simulink model "Sim_8Bus_Chain"  (R2020b)
settings: Solver=FixedStepAuto  StartTime=0  StopTime=3  FixedStep=Ts  RelTol=1e-3
values from neighbouring files (symbols this model uses):
  OtherInputs =     [matlab.mat]
  Ts = 1/Fs    [Main.m]    (also in main.m; matlab.mat = 3.33333333333e-05)
  Wbase = data.basic.Fbase*2*pi    [ConvertExcelFiles.m]    (also in Main.m = Fbase*2*pi; convertExcelFiles.m; main.m = W0; matlab.mat = 376.991118431)
  x_e =     [matlab.mat]
  Zbase = Sbase/Ibase    [Main.m]    (also in matlab.mat = 1e-09)
undefined symbols (not defined in the file or in its folder): DeviceDiscreDamping, DevicePara, DevicePowerFlow, DeviceType
libraries: powerlib x25, SimplexPS x24
settings Model: Creator=admin_user  LastModifiedBy=admin_user

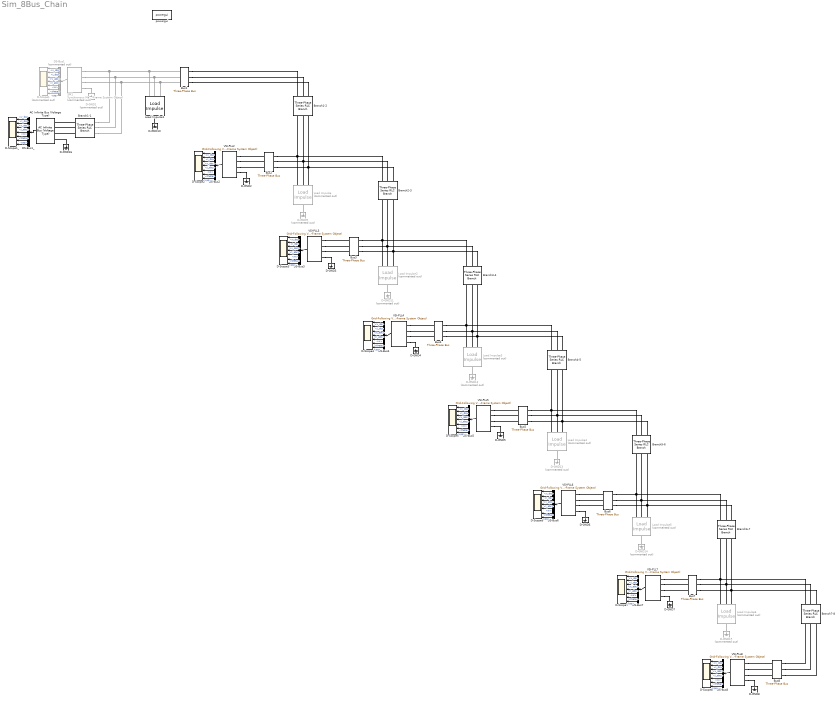
== system Sim_8Bus_Chain ==
  AC Infinite Bus (Voltage Type) : SimplexPS/AC Infinite Bus (Voltage Type)  Ts=Ts  Sbase=Sbase  Vbase=Vbase  Wbase=Wbase  vd=1  vq=0  theta0=0  w=Wbase  R=1e-30
  Branch1-1 : powerlib/Elements/Three-Phase Series RLC Branch  LConnTagsString=A|B|C  RConnTagsString=A|B|C  BranchType=RL  Resistance=(0.001)*Zbase  Inductance=(0.05)*Zbase/Wbase  Capacitance=1e-6  Measurements=None
  Branch1-2 : powerlib/Elements/Three-Phase Series RLC Branch  LConnTagsString=A|B|C  RConnTagsString=A|B|C  BranchType=RL  Resistance=(0.015)*Zbase  Inductance=(0.15)*Zbase/Wbase  Capacitance=1e-6  Measurements=None
  Branch2-3 : powerlib/Elements/Three-Phase Series RLC Branch  LConnTagsString=A|B|C  RConnTagsString=A|B|C  BranchType=RL  Resistance=(0.015)*Zbase  Inductance=(0.15)*Zbase/Wbase  Capacitance=1e-6  Measurements=None
  Branch3-4 : powerlib/Elements/Three-Phase Series RLC Branch  LConnTagsString=A|B|C  RConnTagsString=A|B|C  BranchType=RL  Resistance=(0.015)*Zbase  Inductance=(0.15)*Zbase/Wbase  Capacitance=1e-6  Measurements=None
  Branch4-5 : powerlib/Elements/Three-Phase Series RLC Branch  LConnTagsString=A|B|C  RConnTagsString=A|B|C  BranchType=RL  Resistance=(0.015)*Zbase  Inductance=(0.15)*Zbase/Wbase  Capacitance=1e-6  Measurements=None
  Branch5-6 : powerlib/Elements/Three-Phase Series RLC Branch  LConnTagsString=A|B|C  RConnTagsString=A|B|C  BranchType=RL  Resistance=(0.015)*Zbase  Inductance=(0.15)*Zbase/Wbase  Capacitance=1e-6  Measurements=None
  Branch6-7 : powerlib/Elements/Three-Phase Series RLC Branch  LConnTagsString=A|B|C  RConnTagsString=A|B|C  BranchType=RL  Resistance=(0.015)*Zbase  Inductance=(0.15)*Zbase/Wbase  Capacitance=1e-6  Measurements=None
  Branch7-8 : powerlib/Elements/Three-Phase Series RLC Branch  LConnTagsString=A|B|C  RConnTagsString=A|B|C  BranchType=RL  Resistance=(0.015)*Zbase  Inductance=(0.15)*Zbase/Wbase  Capacitance=1e-6  Measurements=None
  Bus{1..8} (8 alike) : SimplexPS/Three-Phase Bus  Vbase=1  Sbase=1
  D-GND{1,9,11..15} (7 alike) : powerlib/Elements/Ground  Commented=on  LConnTagsString=a
  D-GND{2..8,10,16} (9 alike) : powerlib/Elements/Ground  LConnTagsString=a
  D-Scope1 : Scope  Commented=on  NumInputPorts=7
  D-Scope1_ : Scope  NumInputPorts=7
  D-Scope{2..8} (7 alike) : Scope  NumInputPorts=7
  DS-Bus1 : BusSelector  Commented=on  OutputSignals=v_dq,i_dq,v_abc,i_abc,w,theta,pq
  DS-Bus1_ : BusSelector  OutputSignals=v_dq,i_dq,v_abc,i_abc,w,theta,pq
  DS-Bus{2..8} (7 alike) : BusSelector  OutputSignals=v_dq,i_dq,v_abc,i_abc,w,theta,pq
  Load Impulse{,2..6} (6 alike) : SimplexPS/Load Impulse  Commented=on  t0=1  dt=1/60*4  R=1e-9*Zbase
  Load Impulse1 : SimplexPS/Load Impulse  t0=1  dt=1/60*4  R=1e-9*Zbase
  SM1 : SimplexPS/Synchronous Machine (dq-Frame System Object)  Commented=on  Ts=Ts  Sbase=Sbase  Vbase=Vbase  Wbase=Wbase  DeviceType=DeviceType{1}  DevicePara=DevicePara{1}  PowerFlow=DevicePowerFlow{1}  x0=x_e{1}  OtherInputs=OtherInputs{1}  DiscreMethod=Hybrid Trapezoidal  EnableInsideModification=off  DiscreDampingFlag=on  DiscreDampingValue=DeviceDiscreDamping{1}  LinearizationTimes=1  DirectFeedthrough=off
  VSI-PLL2 : SimplexPS/Grid-Following Voltage-Source Inverter (dq-Frame System Object)  Ts=Ts  Sbase=Sbase  Vbase=Vbase  Wbase=Wbase  DeviceType=DeviceType{2}  DevicePara=DevicePara{2}  PowerFlow=DevicePowerFlow{2}  x0=x_e{2}  OtherInputs=OtherInputs{2}  DiscreMethod=Hybrid Trapezoidal  EnableInsideModification=off  DiscreDampingFlag=on  DiscreDampingValue=DeviceDiscreDamping{2}  LinearizationTimes=1  DirectFeedthrough=off
  VSI-PLL3 : SimplexPS/Grid-Following Voltage-Source Inverter (dq-Frame System Object)  Ts=Ts  Sbase=Sbase  Vbase=Vbase  Wbase=Wbase  DeviceType=DeviceType{3}  DevicePara=DevicePara{3}  PowerFlow=DevicePowerFlow{3}  x0=x_e{3}  OtherInputs=OtherInputs{3}  DiscreMethod=Hybrid Trapezoidal  EnableInsideModification=off  DiscreDampingFlag=on  DiscreDampingValue=DeviceDiscreDamping{3}  LinearizationTimes=1  DirectFeedthrough=off
  VSI-PLL4 : SimplexPS/Grid-Following Voltage-Source Inverter (dq-Frame System Object)  Ts=Ts  Sbase=Sbase  Vbase=Vbase  Wbase=Wbase  DeviceType=DeviceType{4}  DevicePara=DevicePara{4}  PowerFlow=DevicePowerFlow{4}  x0=x_e{4}  OtherInputs=OtherInputs{4}  DiscreMethod=Hybrid Trapezoidal  EnableInsideModification=off  DiscreDampingFlag=on  DiscreDampingValue=DeviceDiscreDamping{4}  LinearizationTimes=1  DirectFeedthrough=off
  VSI-PLL5 : SimplexPS/Grid-Following Voltage-Source Inverter (dq-Frame System Object)  Ts=Ts  Sbase=Sbase  Vbase=Vbase  Wbase=Wbase  DeviceType=DeviceType{5}  DevicePara=DevicePara{5}  PowerFlow=DevicePowerFlow{5}  x0=x_e{5}  OtherInputs=OtherInputs{5}  DiscreMethod=Hybrid Trapezoidal  EnableInsideModification=off  DiscreDampingFlag=on  DiscreDampingValue=DeviceDiscreDamping{5}  LinearizationTimes=1  DirectFeedthrough=off
  VSI-PLL6 : SimplexPS/Grid-Following Voltage-Source Inverter (dq-Frame System Object)  Ts=Ts  Sbase=Sbase  Vbase=Vbase  Wbase=Wbase  DeviceType=DeviceType{6}  DevicePara=DevicePara{6}  PowerFlow=DevicePowerFlow{6}  x0=x_e{6}  OtherInputs=OtherInputs{6}  DiscreMethod=Hybrid Trapezoidal  EnableInsideModification=off  DiscreDampingFlag=on  DiscreDampingValue=DeviceDiscreDamping{6}  LinearizationTimes=1  DirectFeedthrough=off
  VSI-PLL7 : SimplexPS/Grid-Following Voltage-Source Inverter (dq-Frame System Object)  Ts=Ts  Sbase=Sbase  Vbase=Vbase  Wbase=Wbase  DeviceType=DeviceType{7}  DevicePara=DevicePara{7}  PowerFlow=DevicePowerFlow{7}  x0=x_e{7}  OtherInputs=OtherInputs{7}  DiscreMethod=Hybrid Trapezoidal  EnableInsideModification=off  DiscreDampingFlag=on  DiscreDampingValue=DeviceDiscreDamping{7}  LinearizationTimes=1  DirectFeedthrough=off
  VSI-PLL8 : SimplexPS/Grid-Following Voltage-Source Inverter (dq-Frame System Object)  Ts=Ts  Sbase=Sbase  Vbase=Vbase  Wbase=Wbase  DeviceType=DeviceType{8}  DevicePara=DevicePara{8}  PowerFlow=DevicePowerFlow{8}  x0=x_e{8}  OtherInputs=OtherInputs{8}  DiscreMethod=Hybrid Trapezoidal  EnableInsideModification=off  DiscreDampingFlag=on  DiscreDampingValue=DeviceDiscreDamping{8}  LinearizationTimes=1  DirectFeedthrough=off
  powergui : powerlib/powergui  Priority=1  SimulationMode=Discrete  SampleTime=Ts  frequency=60  Iterations=50  frequencyindice=0  Pbase=100e6  ErrMax=1e-4  UnitsV=kV  UnitsW=MW  buscounter=0  FunctionMessages=off  echomessages=off  EnableUseOfTLC=off  CurrentSourceSwitches=off  DisableSnubberDevices=off  DisableRonSwitches=off  DisableVfSwitches=off  DisplayEquations=off  AutomaticDiscreteSolvers=off  SolverType=Tustin/Backward Euler (TBE)  Interpol=off  ExternalGateDelay=off  methode=off  Ts=100  x0status=blocks  SPID=on  SwTol=0  HookPort=off  NonlinearTolerance=1e-4  nMaxIteration=100  ContinueOnMaxIteration=off  RestoreLinks=warning  ResistiveCurrentMeasurement=off  Frange=[0:2:500]  Ylog=off  Xlog=on  ShowGrid=off  save=off  variable=ZData  structure=0  ZoomFFT=off  StartTime=0.0  cycles=1  DisplayStyle=1  fundamental=60  FreqAxis=off  MaxFrequency=1000  frequencyindicesteady=1  RmsSteady=1  display=off
  wires:
  SM1/1 -> DS-Bus1/1
  DS-Bus1/1 -> D-Scope1/1  "<v_dq>"
  DS-Bus1/2 -> D-Scope1/2  "<i_dq>"
  DS-Bus1/3 -> D-Scope1/3  "<v_abc>"
  DS-Bus1/4 -> D-Scope1/4  "<i_abc>"
  DS-Bus1/5 -> D-Scope1/5  "<w>"
  DS-Bus1/6 -> D-Scope1/6  "<theta>"
  DS-Bus1/7 -> D-Scope1/7  "<pq>"
  VSI-PLL2/1 -> DS-Bus2/1
  DS-Bus2/1 -> D-Scope2/1  "<v_dq>"
  DS-Bus2/2 -> D-Scope2/2  "<i_dq>"
  DS-Bus2/3 -> D-Scope2/3  "<v_abc>"
  DS-Bus2/4 -> D-Scope2/4  "<i_abc>"
  DS-Bus2/5 -> D-Scope2/5  "<w>"
  DS-Bus2/6 -> D-Scope2/6  "<theta>"
  DS-Bus2/7 -> D-Scope2/7  "<pq>"
  VSI-PLL3/1 -> DS-Bus3/1
  DS-Bus3/1 -> D-Scope3/1  "<v_dq>"
  DS-Bus3/2 -> D-Scope3/2  "<i_dq>"
  DS-Bus3/3 -> D-Scope3/3  "<v_abc>"
  DS-Bus3/4 -> D-Scope3/4  "<i_abc>"
  DS-Bus3/5 -> D-Scope3/5  "<w>"
  DS-Bus3/6 -> D-Scope3/6  "<theta>"
  DS-Bus3/7 -> D-Scope3/7  "<pq>"
  VSI-PLL4/1 -> DS-Bus4/1
  DS-Bus4/1 -> D-Scope4/1  "<v_dq>"
  DS-Bus4/2 -> D-Scope4/2  "<i_dq>"
  DS-Bus4/3 -> D-Scope4/3  "<v_abc>"
  DS-Bus4/4 -> D-Scope4/4  "<i_abc>"
  DS-Bus4/5 -> D-Scope4/5  "<w>"
  DS-Bus4/6 -> D-Scope4/6  "<theta>"
  DS-Bus4/7 -> D-Scope4/7  "<pq>"
  VSI-PLL5/1 -> DS-Bus5/1
  DS-Bus5/1 -> D-Scope5/1  "<v_dq>"
  DS-Bus5/2 -> D-Scope5/2  "<i_dq>"
  DS-Bus5/3 -> D-Scope5/3  "<v_abc>"
  DS-Bus5/4 -> D-Scope5/4  "<i_abc>"
  DS-Bus5/5 -> D-Scope5/5  "<w>"
  DS-Bus5/6 -> D-Scope5/6  "<theta>"
  DS-Bus5/7 -> D-Scope5/7  "<pq>"
  VSI-PLL6/1 -> DS-Bus6/1
  DS-Bus6/1 -> D-Scope6/1  "<v_dq>"
  DS-Bus6/2 -> D-Scope6/2  "<i_dq>"
  DS-Bus6/3 -> D-Scope6/3  "<v_abc>"
  DS-Bus6/4 -> D-Scope6/4  "<i_abc>"
  DS-Bus6/5 -> D-Scope6/5  "<w>"
  DS-Bus6/6 -> D-Scope6/6  "<theta>"
  DS-Bus6/7 -> D-Scope6/7  "<pq>"
  VSI-PLL7/1 -> DS-Bus7/1
  DS-Bus7/1 -> D-Scope7/1  "<v_dq>"
  DS-Bus7/2 -> D-Scope7/2  "<i_dq>"
  DS-Bus7/3 -> D-Scope7/3  "<v_abc>"
  DS-Bus7/4 -> D-Scope7/4  "<i_abc>"
  DS-Bus7/5 -> D-Scope7/5  "<w>"
  DS-Bus7/6 -> D-Scope7/6  "<theta>"
  DS-Bus7/7 -> D-Scope7/7  "<pq>"
  VSI-PLL8/1 -> DS-Bus8/1
  DS-Bus8/1 -> D-Scope8/1  "<v_dq>"
  DS-Bus8/2 -> D-Scope8/2  "<i_dq>"
  DS-Bus8/3 -> D-Scope8/3  "<v_abc>"
  DS-Bus8/4 -> D-Scope8/4  "<i_abc>"
  DS-Bus8/5 -> D-Scope8/5  "<w>"
  DS-Bus8/6 -> D-Scope8/6  "<theta>"
  DS-Bus8/7 -> D-Scope8/7  "<pq>"
  DS-Bus1_/4 -> D-Scope1_/4  "<i_abc>"
  DS-Bus1_/7 -> D-Scope1_/7  "<pq>"
  DS-Bus1_/3 -> D-Scope1_/3  "<v_abc>"
  DS-Bus1_/1 -> D-Scope1_/1  "<v_dq>"
  DS-Bus1_/5 -> D-Scope1_/5  "<w>"
  AC Infinite Bus (Voltage Type)/1 -> DS-Bus1_/1
  DS-Bus1_/2 -> D-Scope1_/2  "<i_dq>"
  DS-Bus1_/6 -> D-Scope1_/6  "<theta>"
  connections:
  SM1/LConn4 -- D-GND1/LConn1
  VSI-PLL2/LConn4 -- D-GND2/LConn1
  VSI-PLL3/LConn4 -- D-GND3/LConn1
  VSI-PLL4/LConn4 -- D-GND4/LConn1
  VSI-PLL5/LConn4 -- D-GND5/LConn1
  VSI-PLL6/LConn4 -- D-GND6/LConn1
  VSI-PLL7/LConn4 -- D-GND7/LConn1
  VSI-PLL8/LConn4 -- D-GND8/LConn1
  Branch1-2/RConn1 -- Load Impulse/LConn1 -- Bus2/RConn1 -- Branch2-3/LConn1
  Branch1-2/RConn2 -- Load Impulse/LConn2 -- Bus2/RConn2 -- Branch2-3/LConn2
  Branch1-2/RConn3 -- Load Impulse/LConn3 -- Bus2/RConn3 -- Branch2-3/LConn3
  Bus1/RConn1 -- Branch1-2/LConn1
  Bus1/RConn2 -- Branch1-2/LConn2
  Bus1/RConn3 -- Branch1-2/LConn3
  Branch2-3/RConn1 -- Load Impulse2/LConn1 -- Bus3/RConn1 -- Branch3-4/LConn1
  Branch2-3/RConn2 -- Load Impulse2/LConn2 -- Bus3/RConn2 -- Branch3-4/LConn2
  Branch2-3/RConn3 -- Load Impulse2/LConn3 -- Bus3/RConn3 -- Branch3-4/LConn3
  Branch3-4/RConn1 -- Load Impulse3/LConn1 -- Bus4/RConn1 -- Branch4-5/LConn1
  Branch3-4/RConn2 -- Load Impulse3/LConn2 -- Bus4/RConn2 -- Branch4-5/LConn2
  Branch3-4/RConn3 -- Load Impulse3/LConn3 -- Bus4/RConn3 -- Branch4-5/LConn3
  Branch4-5/RConn1 -- Load Impulse4/LConn1 -- Bus5/RConn1 -- Branch5-6/LConn1
  Branch4-5/RConn2 -- Load Impulse4/LConn2 -- Bus5/RConn2 -- Branch5-6/LConn2
  Branch4-5/RConn3 -- Load Impulse4/LConn3 -- Bus5/RConn3 -- Branch5-6/LConn3
  Branch5-6/RConn1 -- Load Impulse5/LConn1 -- Bus6/RConn1 -- Branch6-7/LConn1
  Branch5-6/RConn2 -- Load Impulse5/LConn2 -- Bus6/RConn2 -- Branch6-7/LConn2
  Branch5-6/RConn3 -- Load Impulse5/LConn3 -- Bus6/RConn3 -- Branch6-7/LConn3
  Branch6-7/RConn1 -- Load Impulse6/LConn1 -- Bus7/RConn1 -- Branch7-8/LConn1
  Branch6-7/RConn2 -- Load Impulse6/LConn2 -- Bus7/RConn2 -- Branch7-8/LConn2
  Branch6-7/RConn3 -- Load Impulse6/LConn3 -- Bus7/RConn3 -- Branch7-8/LConn3
  Bus8/RConn1 -- Branch7-8/RConn1
  Bus8/RConn2 -- Branch7-8/RConn2
  Bus8/RConn3 -- Branch7-8/RConn3
  SM1/LConn1 -- Branch1-1/RConn1 -- Load Impulse1/LConn1 -- Bus1/LConn1
  SM1/LConn2 -- Branch1-1/RConn2 -- Load Impulse1/LConn2 -- Bus1/LConn2
  SM1/LConn3 -- Branch1-1/RConn3 -- Load Impulse1/LConn3 -- Bus1/LConn3
  VSI-PLL2/LConn1 -- Bus2/LConn1
  VSI-PLL2/LConn2 -- Bus2/LConn2
  VSI-PLL2/LConn3 -- Bus2/LConn3
  VSI-PLL3/LConn1 -- Bus3/LConn1
  VSI-PLL3/LConn2 -- Bus3/LConn2
  VSI-PLL3/LConn3 -- Bus3/LConn3
  VSI-PLL4/LConn1 -- Bus4/LConn1
  VSI-PLL4/LConn2 -- Bus4/LConn2
  VSI-PLL4/LConn3 -- Bus4/LConn3
  VSI-PLL5/LConn1 -- Bus5/LConn1
  VSI-PLL5/LConn2 -- Bus5/LConn2
  VSI-PLL5/LConn3 -- Bus5/LConn3
  VSI-PLL6/LConn1 -- Bus6/LConn1
  VSI-PLL6/LConn2 -- Bus6/LConn2
  VSI-PLL6/LConn3 -- Bus6/LConn3
  VSI-PLL7/LConn1 -- Bus7/LConn1
  VSI-PLL7/LConn2 -- Bus7/LConn2
  VSI-PLL7/LConn3 -- Bus7/LConn3
  VSI-PLL8/LConn1 -- Bus8/LConn1
  VSI-PLL8/LConn2 -- Bus8/LConn2
  VSI-PLL8/LConn3 -- Bus8/LConn3
  D-GND9/LConn1 -- Load Impulse/RConn1
  D-GND10/LConn1 -- Load Impulse1/RConn1
  D-GND11/LConn1 -- Load Impulse2/RConn1
  D-GND12/LConn1 -- Load Impulse3/RConn1
  D-GND13/LConn1 -- Load Impulse4/RConn1
  D-GND14/LConn1 -- Load Impulse5/RConn1
  D-GND15/LConn1 -- Load Impulse6/RConn1
  Branch1-1/LConn1 -- AC Infinite Bus (Voltage Type)/LConn1
  Branch1-1/LConn2 -- AC Infinite Bus (Voltage Type)/LConn2
  Branch1-1/LConn3 -- AC Infinite Bus (Voltage Type)/LConn3
  D-GND16/LConn1 -- AC Infinite Bus (Voltage Type)/LConn4
